simulink model "zad4"  (R2014b)
settings: Solver=ode45  StartTime=0.0  StopTime=1.8  RelTol=1e-3
values from neighbouring files (symbols this model uses):
  a0 = 0.0636    [zad4_setparam.m]
  a1 = -1.3904    [zad4_setparam.m]
  a2 = 7.576    [zad4_setparam.m]
  b0 = 0.0464    [zad4_setparam.m]
  b1 = -0.3684    [zad4_setparam.m]
  b2 = 0.4496    [zad4_setparam.m]
settings Model: Creator=kuba  LastModifiedBy=kuba
settings DebuggingCC: SolverPrmCheckMsg=none

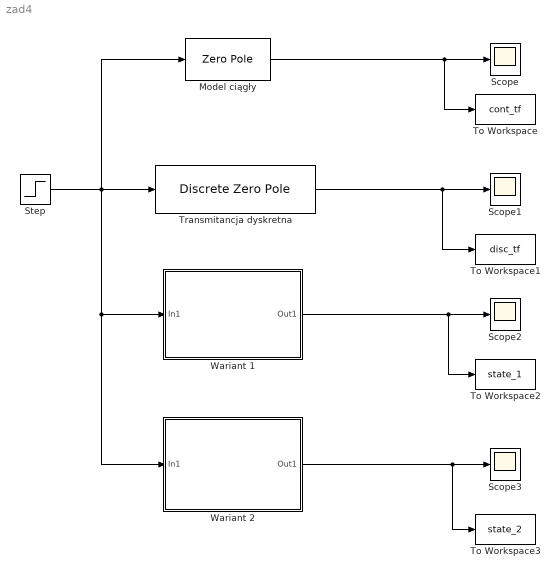
== system zad4 ==
  "Model ciągły " : ZeroPole  Zeros=[-2.5 -7]  Poles=[8 -9 -10]
  Scope{,1..3} (4 alike) : Scope
      Scope2 settings: SaveName=ScopeData2
      Scope3 settings: SaveName=ScopeData3
  Step : Step  SampleTime=0
  To Workspace : ToWorkspace  VariableName=cont_tf  SaveFormat=Timeseries  SampleTime=-1
  To Workspace1 : ToWorkspace  VariableName=disc_tf  SaveFormat=Timeseries  SampleTime=-1
  To Workspace2 : ToWorkspace  VariableName=state_1  SaveFormat=Timeseries  SampleTime=-1
  To Workspace3 : ToWorkspace  VariableName=state_2  SaveFormat=Timeseries  SampleTime=-1
  "Transmitancja dyskretna " : DiscreteZeroPole  Zeros=[0.664 0.1554]  Poles=[7.389 0.105 0.082]  Gain=0.4496  SampleTime=0.25
  "Wariant 1 " : Subsystem
  "Wariant 2 " : Subsystem
  wires:
  Step/1 -> "Wariant 2 "/1(In1), "Wariant 1 "/1(In1), "Model ciągły "/1, "Transmitancja dyskretna "/1
  "Transmitancja dyskretna "/1 -> To Workspace1/1, Scope1/1
  "Model ciągły "/1 -> To Workspace/1, Scope/1
  "Wariant 1 "/1(Out1) -> To Workspace2/1, Scope2/1
  "Wariant 2 "/1(Out1) -> To Workspace3/1, Scope3/1

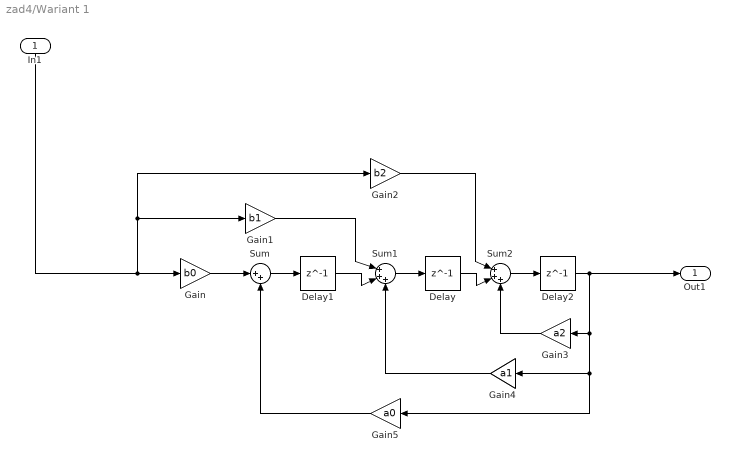
== system zad4/Wariant 1  ==
  In1 : Inport
  Delay : Delay  DelayLength=1  SampleTime=0.25
  Delay1 : Delay  DelayLength=1  SampleTime=0.25
  Delay2 : Delay  DelayLength=1  SampleTime=0.25
  Gain : Gain  Gain=b0
  Gain1 : Gain  Gain=b1
  Gain2 : Gain  Gain=b2
  Gain3 : Gain  Gain=a2
  Gain4 : Gain  Gain=a1
  Gain5 : Gain  Gain=a0
  Sum : Sum  Inputs=|++
  Sum1 : Sum  Inputs=|+++
  Sum2 : Sum  Inputs=|+++
  Out1 : Outport
  wires:
  Gain3/1 -> Sum2/3
  Gain5/1 -> Sum/2
  Gain2/1 -> Sum2/1
  Delay2/1 -> Out1/1, Gain5/1, Gain4/1, Gain3/1
  Delay1/1 -> Sum1/2
  Gain1/1 -> Sum1/1
  Sum2/1 -> Delay2/1
  Sum1/1 -> Delay/1
  Delay/1 -> Sum2/2
  Sum/1 -> Delay1/1
  Gain/1 -> Sum/1
  Gain4/1 -> Sum1/3
  In1/1 -> Gain2/1, Gain1/1, Gain/1

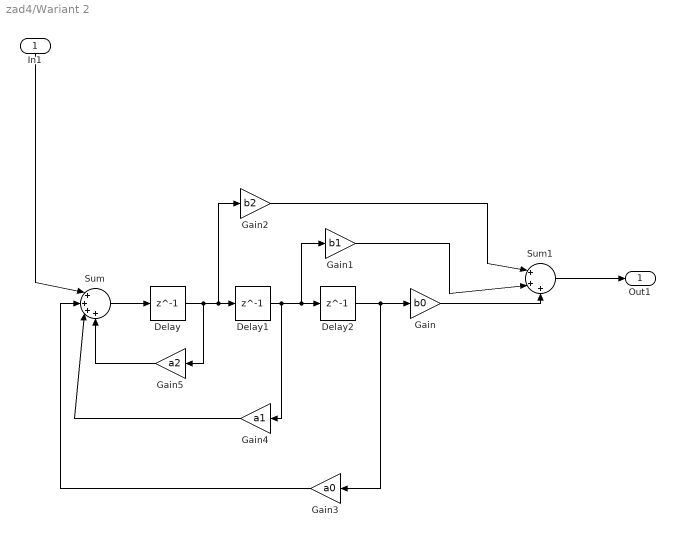
== system zad4/Wariant 2  ==
  In1 : Inport
  Delay : Delay  DelayLength=1  SampleTime=0.25
  Delay1 : Delay  DelayLength=1  SampleTime=0.25
  Delay2 : Delay  DelayLength=1  SampleTime=0.25
  Gain : Gain  Gain=b0
  Gain1 : Gain  Gain=b1
  Gain2 : Gain  Gain=b2
  Gain3 : Gain  Gain=a0
  Gain4 : Gain  Gain=a1
  Gain5 : Gain  Gain=a2
  Sum : Sum  Inputs=|++++
  Sum1 : Sum  Inputs=|+++
  Out1 : Outport
  wires:
  Gain3/1 -> Sum/2
  In1/1 -> Sum/1
  Gain1/1 -> Sum1/2
  Gain5/1 -> Sum/4
  Delay/1 -> Gain5/1, Gain2/1, Delay1/1
  Gain/1 -> Sum1/3
  Sum/1 -> Delay/1
  Sum1/1 -> Out1/1
  Delay1/1 -> Gain4/1, Gain1/1, Delay2/1
  Delay2/1 -> Gain3/1, Gain/1
  Gain4/1 -> Sum/3
  Gain2/1 -> Sum1/1
